simulink model "lqarduino"  (R2022b)
settings: Solver=FixedStepAuto  StartTime=0.0  StopTime=4  RelTol=1e-3  EnableMultiTasking=on
undefined symbols (not defined in the file): C, Cs, DiscIntNeverNeededParam, klq
libraries: arduinolib x2, simulink x1
settings Model: ExtModeTrigDuration=2  Creator=Srikar-PC
settings OptimizationCC: EnhancedBackFolding=on  PassReuseOutputArgsAs=Individual arguments  ZeroExternalMemoryAtStartup=off  ZeroInternalMemoryAtStartup=off  MaxStackSize=64  OptimizeBlockOrder=speed  DifferentSizesBufferReuse=on  OptimizationCustomize=off  EfficientTunableParamExpr=on
settings DebuggingCC: ParameterTunabilityLossMsg=error
settings HardwareCC: ProdBitPerInt=16  ProdBitPerPointer=16  ProdBitPerSizeT=16  ProdBitPerPtrDiffT=16  ProdLargestAtomicFloat=None  ProdWordSize=8  ProdHWDeviceType=Atmel->AVR  UseEmbeddedCoderFeatures=off  UseSimulinkCoderFeatures=off
settings SFSimCC: MATLABDynamicMemAlloc=off
settings RTWCC: Description=Embedded Coder  SystemTargetFile=ert.tlc  HardwareBoard=Arduino Uno  TLCOptions=-aInlineSetEventsForThisBaseRateFcn=TLC_FALSE -aSuppressMultiTaskScheduler=TLC_FALSE -aRateBasedStepFcn=1  TemplateMakefile=ert_default_tmf  Toolchain=Arduino AVR  BuildConfiguration=Faster Runs
settings CodeAppCC: ForceParamTrailComments=on  IgnoreCustomStorageClasses=off  OperatorAnnotations=on  SimulinkDataObjDesc=on  SFDataObjDesc=on  InsertBlockDesc=on
settings ERTTargetCC: SupportContinuousTime=on  SupportNonInlinedSFcns=on  SupportVariableSizeSignals=on  ExtModeTransport=3  ExtModeStaticAlloc=on  ExtModeAutomaticAllocSize=off  ExtModeStaticAllocSize=250  ExtModeMexFile=ext_xcp  ExtModeIntrfLevel=Level2 - Open

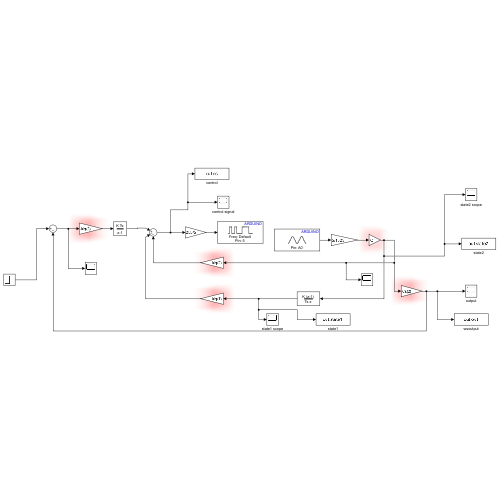
[thumbnail: Simulink's stored preview of the top-level diagram]
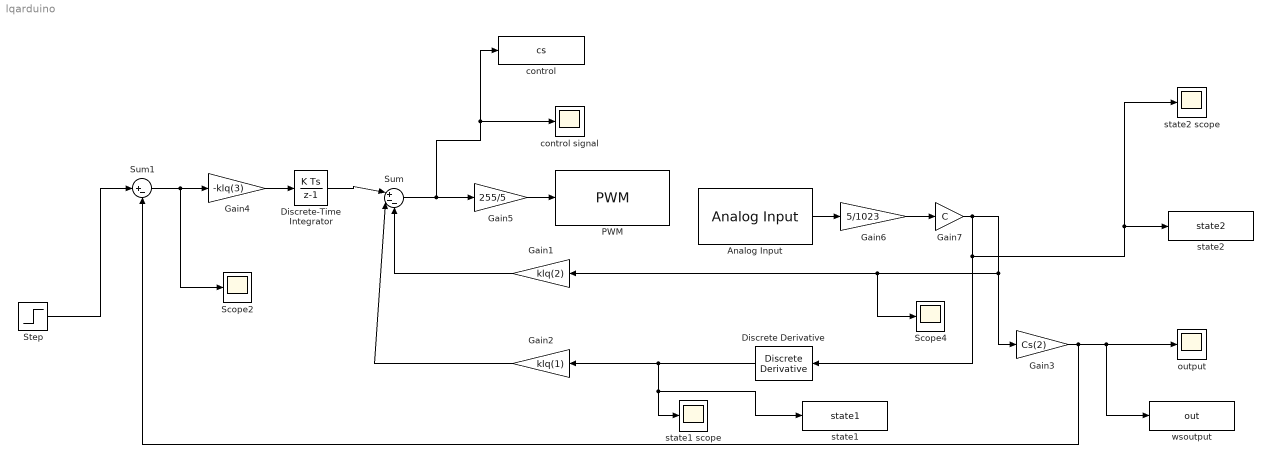
== system lqarduino ==
  Analog Input : arduinolib/Analog Input  pinNumber=0  ReadResultsOnly=off  ConversionTriggerSource=Software  ExternalTriggerType=uint32( 0 )  OutputDataType=uint16  EnableConversionCompleteNotify=off  EnableOuputStatus=off  SampleTime=0.01  blockPlatform=arduino
  Discrete Derivative : simulink/Discrete/Discrete Derivative  gainval=1  ICPrevScaledInput=0  OutMin=[]  OutMax=[]  OutDataTypeStr=double  OutputDataTypeScalingMode=double  OutDataType=fixdt(1, 16)  OutScaling=2^-10  DoSatur=off
  Discrete-Time Integrator : DiscreteIntegrator  SampleTime=0.01  OutDataTypeStr=double  ICPrevOutput=DiscIntNeverNeededParam  ICPrevScaledInput=DiscIntNeverNeededParam
  Gain1 : Gain  Gain=klq(2)
  Gain2 : Gain  Gain=klq(1)
  Gain3 : Gain  Gain=Cs(2)
  Gain4 : Gain  Gain=-klq(3)  OutDataTypeStr=double
  Gain5 : Gain  Gain=255/5
  Gain6 : Gain  Gain=5/1023
  Gain7 : Gain  Gain=C
  PWM : arduinolib/PWM  pinNumber=5  frequencyType=Default  desiredFrequency=490.2  achievableFrequency=490.2
  Scope2 : Scope
  Scope4 : Scope
  Step : Step  SampleTime=0.01
  Sum : Sum  Inputs=|+--
  Sum1 : Sum  Inputs=|+-
  control : ToWorkspace  VariableName=cs  SampleTime=0.01
  control signal : Scope
  output : Scope
  state1 : ToWorkspace  VariableName=state1  SampleTime=0.01
  state1 scope : Scope
  state2 : ToWorkspace  VariableName=state2  SampleTime=0.01
  state2 scope : Scope
  wsoutput : ToWorkspace  VariableName=out  SampleTime=0.01
  wires:
  Gain1/1 -> Sum/3
  Gain3/1 -> Sum1/2, wsoutput/1, output/1
  Gain2/1 -> Sum/2
  Discrete-Time Integrator/1 -> Sum/1
  Sum1/1 -> Scope2/1, Gain4/1
  Step/1 -> Sum1/1
  Gain4/1 -> Discrete-Time Integrator/1
  Sum/1 -> control/1, control signal/1, Gain5/1
  Gain5/1 -> PWM/1
  Analog Input/1 -> Gain6/1
  Gain6/1 -> Gain7/1
  Discrete Derivative/1 -> state1/1, state1 scope/1, Gain2/1
  Gain7/1 -> state2 scope/1, state2/1, Discrete Derivative/1, Gain3/1, Scope4/1, Gain1/1
